simulink model "example_Fuel"  (R2018b)
settings: Solver=ode45  StartTime=0.0  StopTime=10.0  RelTol=1e-3  EnableMultiTasking=on
undefined symbols (not defined in the file): path_carnot
libraries: carnot x4
settings Model: Creator=drhf  LastModifiedBy=drhf
settings DataIOCC: LimitDataPoints=on  SaveFormat=Array
settings OptimizationCC: DefaultParameterBehavior=Inlined  LifeSpan=inf
settings DebuggingCC: UnderspecifiedInitializationDetection=Classic  MergeDetectMultiDrivingBlocksExec=none  SolverPrmCheckMsg=warning  SFUnexpectedBacktrackingDiag=warning  SFNoUnconditionalDefaultTransitionDiag=warning  SFExecutionAtInitializationDiag=none
settings HardwareCC: ProdBitPerPointer=32  ProdBitPerSizeT=32  ProdBitPerPtrDiffT=32  ProdLargestAtomicFloat=None  ProdIntDivRoundTo=Undefined  ProdEndianess=Unspecified  ProdWordSize=32  ProdHWDeviceType=32-bit Generic
settings ModelReferenceCC: PropagateSignalLabelsOutOfModel=off
settings SFSimCC: SimUseLocalCustomCode=off
settings RTWCC: RTWUseLocalCustomCode=off
settings CodeAppCC: StateflowObjectComments=on
settings GRTTargetCC: TargetLangStandard=C89/C90 (ANSI)  GeneratePreprocessorConditionals=Disable all
settings ConfigComp: CovMetricSettings=dw  CovHtmlReporting=on  CovSaveCumulativeToWorkspaceVar=on  CovSaveSingleToWorkspaceVar=on  CovExternalEMLEnable=off

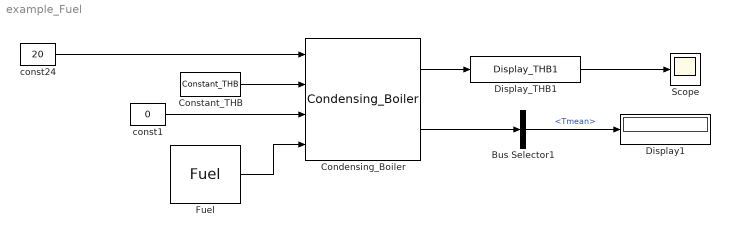
== system example_Fuel ==
  Bus Selector1 : BusSelector  OutputSignals=Tmean
  Condensing_Boiler : carnot/Source/Boiler/Condensing_Boiler  Tini=20  PathName=fullfile(path_carnot('libsl'), 'Source', 'Boiler', 'Condensing_Boiler', 'parameter_set')  FileName='CondensingBoiler_20kW.mat'  userPath=off  userParam=off  Pgas=20000  HeatLoss=2.5  Volume=0.0035  whichTforEfficiency=mean of inlet and outlet temperature  TableRelativePower=[0 0.1 1]  TableTemperatures=[10 50 90]  TableData=[1 1 1; 1.08 0.92 0.85; 1.06 0.9 0.83]  ElectricPower=[0 50 200]  relQdotMin=0.1  dplin=10  dpqua=100  nodes=3
  Constant_THB : carnot/Source/Simple/Constant_THB  t=40  mdot=0  p=1e5  mID=No Pressure Drop  fluid=Water  mix=0  mix2=0  mix3=0  dia=0.02  hgt=0
  Display1 : Display
  Display_THB1 : carnot/Outputs/Display_THB1  t=on  m=off  p=off  id=off  mix=off  d=off
  Fuel : carnot/Source/Energy/Fuel  Temperature=20  Pressure=101300  PathName=fullfile(path_carnot('libsl'), 'Source', 'Energy', 'Fuel', 'parameter_set')  FileName='DefaultFuel_Gas.mat'  userPath=off  userParam=off  ft=1  stoichAir=3.5  combustion_enthalpy=[51400000 56900000]  Tcondensation=[45 25]  massfraction=[0.33 0.67 0 0 0 0]  price=1
  Scope : Scope
  const1 : Constant  Value=0
  const24 : Constant  Value=20
  wires:
  Fuel/1 -> Condensing_Boiler/4
  Constant_THB/1 -> Condensing_Boiler/2
  const24/1 -> Condensing_Boiler/1
  const1/1 -> Condensing_Boiler/3
  Condensing_Boiler/1 -> Display_THB1/1
  Display_THB1/1 -> Scope/1
  Condensing_Boiler/2 -> Bus Selector1/1
  Bus Selector1/1 -> Display1/1  "<Tmean>"
